simulink model "modelo"  (R2023a)
settings: Solver=ode45  StartTime=0.0  StopTime=10.0  MaxStep=0.2  RelTol=1e-3
model workspace: external: MATLAB File C:\Users\pinki\OneDrive\aviãozinho\monociclo\numvars.m (data not in the file)
values from neighbouring files (symbols this model uses):
  pos0 = [0.05; 0.1; 0.004; 0.07]    [numvars.m]
  vel0 = [0; 0; 0; 0]    [numvars.m]
settings Model: Creator=pinki  LastModifiedBy=pinki
settings DataIOCC: InspectSignalLogs=on

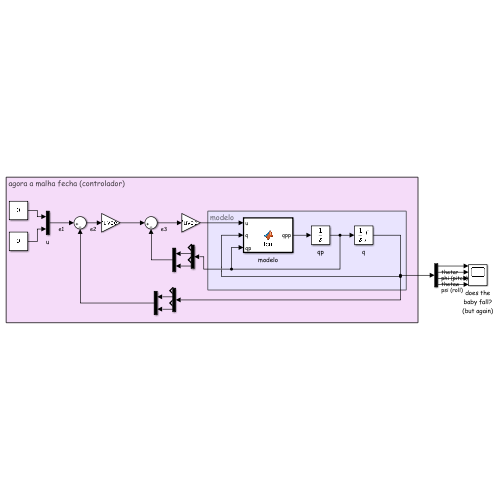
[thumbnail: Simulink's stored preview of the top-level diagram]
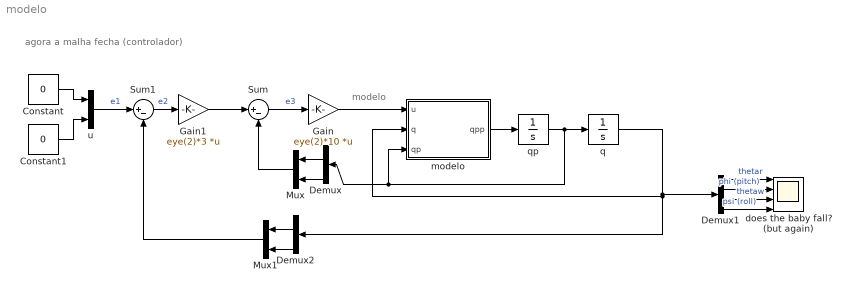
== system modelo ==
  note: modelo
  note: agora a malha fecha (controlador)
  Constant : Constant  Value=0
  Constant1 : Constant  Value=0
  Demux : Demux
  Demux1 : Demux
  Demux2 : Demux
  Gain : Gain  Gain=eye(2)*10  Multiplication=Matrix(K*u) (u vector)
  Gain1 : Gain  Gain=eye(2)*3  Multiplication=Matrix(K*u) (u vector)
  Mux : Mux  Inputs=2
  Mux1 : Mux  Inputs=2
  Sum : Sum  Inputs=|+-
  Sum1 : Sum  Inputs=|+-
  does the baby fall? (but again) : Scope  NumInputPorts=4
  modelo : MATLAB Function  Description=nonlinear model  TreatAsAtomicUnit=on
  q : Integrator  InitialCondition=pos0  LimitOutput=on  UpperSaturationLimit=[inf; pi/2; inf; pi/2]  LowerSaturationLimit=-[inf; pi/2; inf; pi/2]  ContinuousStateAttributes='q'
  qp : Integrator  InitialCondition=vel0  ContinuousStateAttributes='qp'
  u : Mux  Inputs=2
  wires:
  Sum/1 -> Gain/1  "e3"
  modelo/1(qpp) -> qp/1
  Sum1/1 -> Gain1/1  "e2"
  u/1 -> Sum1/1  "e1"
  qp/1 -> modelo/3(qp), Demux/1, q/1
  Demux1/1 -> does the baby fall? (but again)/1  "thetar"
  Demux1/2 -> does the baby fall? (but again)/2  "phi (pitch)"
  Demux1/3 -> does the baby fall? (but again)/3  "thetaw"
  Demux1/4 -> does the baby fall? (but again)/4  "psi (roll)"
  Demux/2 -> Mux/1
  Demux/4 -> Mux/2
  Mux/1 -> Sum/2
  Demux2/4 -> Mux1/2
  Mux1/1 -> Sum1/2
  q/1 -> Demux2/1, modelo/2(q), Demux1/1
  Demux2/2 -> Mux1/1
  Constant/1 -> u/1
  Constant1/1 -> u/2
  Gain/1 -> modelo/1(u)
  Gain1/1 -> Sum/1

== matlab function modelo/modelo ==
  data: qpp output; u input; q input; qp input
function qpp = fcn(u,q,qp)
qpp = zeros(4,1);

mono = monociclo;
psi = q(4);
psip = qp(4);

phi = q(2);
phip = qp(2);

thetar = q(1);
thetarp = qp(1);

thetaw = q(3);
thetawp = qp(4);

m11 = mono.jr;
m12 = m11;
m21 = m11;
m22 = (mono.jbw+mono.jr+(mono.mb+mono.mr+mono.mw)*mono.rw^2 ...
+2*(mono.l*(mono.mb*mono.rw+mono.mr*mono.rw)+mono.mr*mono.rw*mono.d)*cos(psi)...
+(mono.l^2*(mono.mb+mono.mr)+mono.mr*mono.d^2+2*mono.l*mono.mr*mono.d)*cos(psi)^2);
m33 = mono.jw+(mono.mb+mono.mr+mono.mw)*mono.rw^2;
m34 = mono.rw*cos(psi)*(mono.mr*mono.d+mono.l*mono.mb+mono.l*mono.mr);
m43 = m34;
m44 = mono.jbr+mono.mb*mono.l^2+mono.mr*mono.l^2+mono.mr*mono.d^2 ...
    +2*mono.l*mono.mr*mono.d;

M = zeros(4,4);
    M(1,1) = m11;
    M(1,2) = m12;
    M(2,1) = m21;
    M(2,2) = m22;
    M(3,3) = m33;
    M(3,4) = m34;
    M(4,3) = m43;
    M(4,4) = m44;

v1 = (mono.ker*mono.ktr*mono.nr*(mono.nr*thetarp))/mono.rer ...
     - mono.bvr*thetar;
v2 = -(mono.ker*mono.ktr*mono.nr*(mono.nr*thetarp))/mono.rer ...
     - 2*(mono.l*mono.mb+mono.mr*mono.d)*mono.rw*phip*psip*sin(psi) ...
     - (mono.mr*mono.l^2+mono.mb*mono.l^2+mono.mr*mono.d^2+2*mono.l*mono.mr*mono.d)*phip*psip*sin(2*psi) ...
     - mono.bvr*thetar;
v3 = (mono.ker*mono.ktw*mono.nw*(mono.nw*thetawp-psip))/mono.rew ...
    + (mono.l*mono.mb+mono.d*mono.mr+mono.l*mono.mr)*mono.rw*psip^2*sin(psi) ...
    + mono.bvw*thetaw;
v4 = -(mono.ker*mono.ktw*mono.nw*(mono.nw*thetawp-psip))/mono.rew ...
    + (mono.l*mono.mb+mono.d*mono.mr+mono.l*mono.mr)*mono.rw*phip^2*sin(psi) ...
    + (sin(2*psi)*phip^2*((mono.mb*mono.l^2)+(mono.mr*mono.l^2) ...
    + (mono.mr*mono.d^2))/2+mono.l*mono.mr*mono.d)+mono.bvw*thetaw;

V = zeros(4,1);
    V(1) = v1;
    V(2) = v2;
    V(3) = v3;
    V(4) = v4;

g2 = -mono.g*sin(phi)*((mono.mb+mono.mr+mono.mw)*mono.rw+(mono.l*mono.mb ...
    + mono.l*mono.mr + mono.mr*mono.d)*cos(psi));
g4 = -mono.g*cos(phi)*sin(psi)*(mono.mr*mono.d+mono.l*mono.mb+mono.l*mono.mr);

G = zeros(4,1);
    G(2) = g2;
    G(4) = g4;

p11 = (12*mono.ktr*mono.nr)/mono.rr;
p12 = -p11;
p23 = (12*mono.ktw*mono.nw)/mono.rw;
p24 = -p23;

P = zeros(4,2);
    P(1,1) = p11;
    P(2,1) = p12;
    P(3,2) = p23;
    P(4,2) = p24;
    
qpp = M\(-V-G+P*u);
